simulink model "FW_IEEEIA"  (R2018b)
settings: Solver=ode45  StartTime=0.0  StopTime=30  FixedStep=Ts  RelTol=1e-4  EnableMultiTasking=on
InitFcn:
  | Ts = 1e-4;
  | 
  | 
  | Rs = 0.8975;
  | Ld = 15e-3;
  | Lq = 19e-3;
  | Pn = 3;
  | flux = 0.1764;
  | 
  | 
  | %ASR coef
  | kp_speed = 0.01;
  | ki_speed = 0.01*50;
  | 
  | kp_comp = 0.65;
  | ki_comp = 0.001*pi*kp_comp;
  | 
  | 
  | %FW coef
  | kpd_FW = 2;
  | kid_FW = 0.1;
  | 
  | 
  | %ACR coef
  | kp_cur = Lq*375;
  | ki_cur = Rs*375;
undefined symbols (not defined in the file or in its folder): DiscIntNeverNeededParam
libraries: powerlib x5, simulink x4, powerlib_extras x2
settings Model: Creator=SUN  LastModifiedBy=liangjin
settings SolverCC: ZeroCrossControl=DisableAll
settings DataIOCC: LimitDataPoints=on  SaveFormat=Array
settings OptimizationCC: ExpressionDepthLimit=2147483647  InitFltsAndDblsToZero=on  LifeSpan=inf
settings DebuggingCC: UnderspecifiedInitializationDetection=Classic  MergeDetectMultiDrivingBlocksExec=none  SolverPrmCheckMsg=warning  FcnCallInpInsideContextMsg=warning  StateNameClashWarn=warning  SFUnexpectedBacktrackingDiag=warning  SFNoUnconditionalDefaultTransitionDiag=warning  SFExecutionAtInitializationDiag=none
settings HardwareCC: ProdBitPerPointer=32  ProdBitPerSizeT=32  ProdBitPerPtrDiffT=32  ProdLargestAtomicFloat=None  ProdIntDivRoundTo=Undefined  ProdEndianess=Unspecified  ProdWordSize=32  ProdHWDeviceType=32-bit Generic
settings ModelReferenceCC: PropagateSignalLabelsOutOfModel=off
settings SFSimCC: SimUseLocalCustomCode=off
settings RTWCC: RTWUseLocalCustomCode=off
settings CodeAppCC: StateflowObjectComments=on
settings GRTTargetCC: TargetLangStandard=C89/C90 (ANSI)  CombineOutputUpdateFcns=off  GRTInterface=on
settings ConfigComp: CovMetricSettings=dw  CovHtmlReporting=on  CovSaveCumulativeToWorkspaceVar=on  CovSaveSingleToWorkspaceVar=on  CovExternalEMLEnable=off  CovSFcnEnable=off
settings SimscapeCC: SimscapeNormalizeSystem=off

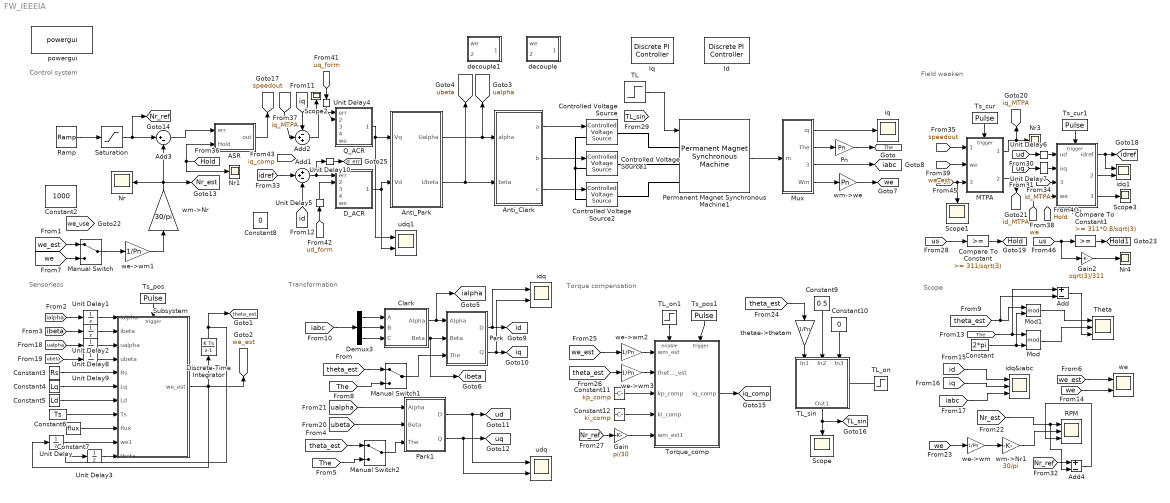
== system FW_IEEEIA ==
  note: Field weaken
  note: Control system
  note: Torque compensation
  note: Scope
  note: Transformation
  note: Sensorless
  ASR : Subsystem
  Add : Sum  Inputs=+-
  Add1 : Sum  Inputs=++-
  Add2 : Sum  Inputs=-++
  Add3 : Sum  Inputs=|+-
  Add4 : Sum  Inputs=+-
  Anti_Clark : Subsystem
  Anti_Park : Subsystem
  Clark : Subsystem
  Compare To Constant : simulink/Logic and Bit Operations/Compare To Constant  relop=>=  const=311/sqrt(3)  OutDataTypeStr=boolean
  Compare To Constant1 : simulink/Logic and Bit Operations/Compare To Constant  relop=>=  const=311*0.8/sqrt(3)  OutDataTypeStr=boolean
  Constant : Constant  Value=2*pi
  Constant10 : Constant  Value=0
  Constant11 : Constant  Value=kp_comp
  Constant12 : Constant  Value=ki_comp
  Constant2 : Constant  Value=1000
  Constant3 : Constant  Value=Rs
  Constant4 : Constant  Value=Lq
  Constant5 : Constant  Value=Ld
  Constant6 : Constant  Value=Ts
  Constant7 : Constant  Value=flux
  Constant8 : Constant  Value=0
  Constant9 : Constant  Value=0.5
  Controlled Voltage Source : powerlib/Electrical Sources/Controlled Voltage Source  Initialize=on  Source_Type=AC  Amplitude=0  Phase=0  Frequency=0  Measurements=Voltage
  Controlled Voltage Source1 : powerlib/Electrical Sources/Controlled Voltage Source  Initialize=on  Source_Type=AC  Amplitude=0  Phase=0  Frequency=0  Measurements=Voltage
  Controlled Voltage Source2 : powerlib/Electrical Sources/Controlled Voltage Source  Initialize=on  Source_Type=AC  Amplitude=0  Phase=0  Frequency=0  Measurements=Voltage
  D_ACR : Subsystem
  Demux3 : Demux  Outputs=3
  Discrete-Time Integrator : DiscreteIntegrator  gainval=1  SampleTime=Ts  ICPrevOutput=DiscIntNeverNeededParam  ICPrevScaledInput=DiscIntNeverNeededParam
  FW : Subsystem
  Gain : Gain  Gain=pi/30
  Gain2 : Gain  Gain=sqrt(3)/311
  Id : powerlib_extras/Discrete  Control Blocks/Discrete PI Controller  Kp=Ld*375  Ki=Rs*375  Par_Limits=[311*sqrt(1/3) -311*sqrt(1/3)]  Init=0  Ts=Ts
  Iq : powerlib_extras/Discrete  Control Blocks/Discrete PI Controller  Kp=Lq*375  Ki=Rs*375  Par_Limits=[311*sqrt(1/3) -311*sqrt(1/3)]  Init=0  Ts=Ts
  MTPA : Subsystem
  Manual Switch : ManualSwitch
  Manual Switch1 : ManualSwitch
  Manual Switch2 : ManualSwitch
  Mod : Math  Operator=mod  SaturateOnIntegerOverflow=on
  Mod1 : Math  Operator=mod  SaturateOnIntegerOverflow=on
  Mux : Subsystem
  Nr{,1,3..4} (4 alike) : Scope
  Park : Subsystem
  Park1 : Subsystem
  Permanent Magnet Synchronous Machine1 : powerlib/Machines/Permanent Magnet Synchronous Machine  NbPhases=3  FluxDistribution=Sinusoidal  RotorType=Salient-pole  MechanicalLoad=Torque Tm  PresetModel=No  ShowDetailedParameters=on  MeasurementBus=off  Resistance=0.8975  Inductance=8.5e-3  dqInductances=[15e-3,19e-3]  La=0.000835  MachineConstant=Flux linkage established by magnets (V.s)  Flux=0.1764  VoltageCst=95.9863  TorqueCst=0.7938  Flat=120  Mechanical=[0.000311 0.0000001 3 0]  PolePairs=3  InitialConditions=[0,0, 0,0]  InitialConditions5ph=[0 0 0 0 0 0]  TsPowergui=0  TsBlock=Ts  RefAngle=Aligned with phase A axis (original Park)
  Pn : Gain  Gain=Pn
  Q_ACR : Subsystem
  RPM : Scope  NumInputPorts=3
  Ramp : simulink/Sources/Ramp  slope=500  start=0  InitialOutput=0
  Saturation : Saturate  UpperLimit=6000  LowerLimit=-1000
  Scope{,1..3} (4 alike) : Scope
  Subsystem : Subsystem
  TL : Step  Time=5  After=0  SampleTime=Ts
  TL_on : Step  Time=5  SampleTime=0
  TL_on1 : Step  Time=5  SampleTime=0
  TL_sin : Subsystem
  Theta : Scope  NumInputPorts=3
  Torque_comp : Subsystem
  Ts_cur : DiscretePulseGenerator  PulseType=Time based  Period=Ts  PulseWidth=50
  Ts_cur1 : DiscretePulseGenerator  PulseType=Time based  Period=Ts  PulseWidth=50
  Ts_pos : DiscretePulseGenerator  PulseType=Time based  Period=Ts  PulseWidth=50
  Ts_pos1 : DiscretePulseGenerator  PulseType=Time based  Period=Ts  PulseWidth=50
  Unit Delay{,1..10} (11 alike) : UnitDelay  SampleTime=Ts
  decouple : Subsystem
  decouple1 : Subsystem
  idq : Scope  NumInputPorts=2
  idq&iabc : Scope  NumInputPorts=3
  idq1 : Scope  NumInputPorts=2
  iq : Scope
  powergui : powerlib/powergui  SimulationMode=Discrete  SampleTime=1e-5  frequency=60  Iterations=50  frequencyindice=0  Pbase=100e6  ErrMax=1e-4  UnitsV=kV  UnitsW=MW  buscounter=0  FunctionMessages=off  echomessages=off  EnableUseOfTLC=off  CurrentSourceSwitches=off  DisableSnubberDevices=off  DisableRonSwitches=off  DisableVfSwitches=off  DisplayEquations=off  SolverType=Tustin/Backward Euler (TBE)  Interpol=off  ExternalGateDelay=off  methode=off  Ts=100  x0status=blocks  SPID=off  SwTol=0  HookPort=off  RestoreLinks=warning  ResistiveCurrentMeasurement=off  Frange=[0:2:500]  Ylog=off  Xlog=on  ShowGrid=off  save=off  variable=ZData  structure=idq  ZoomFFT=off  StartTime=0.0  cycles=1  DisplayStyle=1  fundamental=60  FreqAxis=off  MaxFrequency=1000  frequencyindicesteady=1  RmsSteady=1  display=off
  thetae->thetam : Gain  Gain=1/Pn
  udq : Scope  NumInputPorts=2
  udq1 : Scope  NumInputPorts=2
  we : Scope  NumInputPorts=2
  we->wm{,1..3} (4 alike) : Gain  Gain=1/Pn
  wm->Nr : Gain  Gain=30/pi
  wm->Nr1 : Gain  Gain=30/pi
  wm->we : Gain  Gain=Pn
  tag scope: Hold1=global, Hold=global, Nr_est=global, Nr_ref=global, TL_sin=global, The=global, d_err=global, iabc=global, ialpha=global, ibeta=global, id=global, id_MTPA=global, idref=global, iq=global, iq_MTPA=global, iq_comp=global, speedout=global, theta_est=global, ualpha=global, ubeta=global, ud=global, uq=global, we=global, we_est=global, we_use=global
  wires:
  Permanent Magnet Synchronous Machine1/1 -> Mux/1(m)
  Add3/1 -> ASR/1(err)
  wm->Nr/1 -> [Nr_est], Add3/2, Nr/1
  Mux/1(iq) -> iq/1
  Mux/2(The) -> Pn/1
  Pn/1 -> [The]
  Mux/4(Wm) -> wm->we/1
  Mux/3(Iabc) -> [iabc]
  Clark/1(Alpha) -> [ialpha], Park/1(Alpha)
  Demux3/1 -> Clark/1(A)
  Demux3/2 -> Clark/2(B)
  Demux3/3 -> Clark/3(C)
  Clark/2(Beta) -> Park/2(Beta), [ibeta]
  Anti_Clark/2(b) -> Controlled Voltage Source1/1
  Anti_Clark/3(c) -> Controlled Voltage Source2/1
  Constant/1 -> Mod1/2, Mod/2
  Mod/1 -> Theta/2
  wm->we/1 -> [we]
  Ramp/1 -> Saturation/1
  we->wm1/1 -> wm->Nr/1
  Anti_Park/1(Ualpha) -> Anti_Clark/1(alpha), [ualpha]
  Anti_Park/2(Ubeta) -> Anti_Clark/2(beta), [ubeta]
  [we_est] -> we/1
  [we_est] -> Manual Switch/1
  [we] -> Manual Switch/2
  [theta_est] -> Manual Switch1/1
  [The] -> Manual Switch1/2
  Park/1(D) -> idq/1, [id]
  Park/2(Q) -> [iq], idq/2
  [The] -> Add/1, Mod/1
  [id] -> idq&iabc/1
  [iq] -> idq&iabc/2
  [iabc] -> idq&iabc/3
  [id] -> Add1/3
  [iq] -> Add2/1
  [The] -> Manual Switch2/2
  [theta_est] -> Manual Switch2/1
  [ubeta] -> Park1/2(Beta)
  [ualpha] -> Park1/1(Alpha)
  Park1/1(D) -> [ud], udq/1
  Park1/2(Q) -> udq/2, [uq]
  Constant3/1 -> Subsystem/5(Rs)
  Constant4/1 -> Subsystem/6(Lq)
  Constant5/1 -> Subsystem/7(Ld)
  Constant6/1 -> Subsystem/8(Ts)
  Constant7/1 -> Subsystem/9(flux)
  Unit Delay/1 -> Subsystem/10(we1)
  Ts_pos/1 -> Subsystem/Trigger
  Unit Delay3/1 -> Subsystem/11(theta)
  [theta_est] -> Add/2, Mod1/1
  Mod1/1 -> Theta/1
  [iabc] -> Demux3/1
  Discrete-Time Integrator/1 -> Unit Delay3/1, [theta_est]
  Anti_Clark/1(a) -> Controlled Voltage Source/1
  [we] -> we->wm/1
  we->wm/1 -> wm->Nr1/1
  wm->Nr1/1 -> RPM/2
  [Nr_est] -> Add4/2, RPM/1
  Ts_cur/1 -> MTPA/Trigger
  [we] -> we/2
  [theta_est] -> thetae->thetam/1
  thetae->thetam/1 -> TL_sin/1(In1)
  Constant9/1 -> TL_sin/2(In2)
  Constant10/1 -> TL_sin/3(In3)
  TL_on/1 -> TL_sin/Enable
  TL_sin/1(Out1) -> [TL_sin], Scope/1
  we->wm2/1 -> Torque_comp/1(wm_est)
  we->wm3/1 -> Torque_comp/2(thetam_est)
  Constant11/1 -> Torque_comp/3(kp_comp)
  Constant12/1 -> Torque_comp/4(ki_comp)
  Torque_comp/1(iq_comp) -> [iq_comp]
  [Nr_ref] -> Gain/1
  Gain/1 -> Torque_comp/5(wm_est1)
  Ts_pos1/1 -> Torque_comp/Trigger
  TL_on1/1 -> Torque_comp/Enable
  [we_est] -> we->wm2/1
  [theta_est] -> we->wm3/1
  Ts_cur1/1 -> FW/Trigger
  [speedout] -> MTPA/1(speedout)
  Add/1 -> Theta/3
  MTPA/1(iq_MTPA) -> Nr3/1, [iq_MTPA]
  MTPA/2(id_MTPA) -> [id_MTPA]
  [idref] -> Add1/2
  [Nr_ref] -> Add4/1
  Add4/1 -> RPM/3
  [id_MTPA] -> FW/3(id_MTPA)
  Saturation/1 -> Add3/1, [Nr_ref]
  ASR/1(out) -> [speedout]
  [iq_MTPA] -> Add2/2
  [us] -> Compare To Constant/1
  Compare To Constant/1 -> [Hold]
  [we] -> FW/4(we)
  [we_est] -> MTPA/2(we)
  FW/1(idref) -> [idref], idq1/1
  [uq_form] -> Unit Delay4/1
  Unit Delay4/1 -> Q_ACR/2(uq_form)
  [ud_form] -> Unit Delay5/1
  Unit Delay5/1 -> D_ACR/2(ud_form)
  FW/2(piout) -> idq1/2
  Add2/1 -> Scope2/1, Q_ACR/1(err)
  Add1/1 -> Unit Delay10/1, D_ACR/1(err)
  Q_ACR/1(iqout) -> udq1/1, Anti_Park/1(Vq)
  D_ACR/1(idout) -> Anti_Park/2(Vd), udq1/2
  [ud] -> Unit Delay6/1
  Unit Delay6/1 -> FW/1(ud)
  [uq] -> Unit Delay7/1
  Unit Delay7/1 -> FW/2(uq)
  [us] -> Gain2/1, Compare To Constant1/1
  Gain2/1 -> Nr4/1
  Compare To Constant1/1 -> [Hold1]
  Subsystem/1(we_est) -> [we_est], Discrete-Time Integrator/1, Unit Delay/1
  [ualpha] -> Unit Delay8/1
  [ubeta] -> Unit Delay9/1
  [ialpha] -> Unit Delay1/1
  [ibeta] -> Unit Delay2/1
  Manual Switch/1 -> we->wm1/1
  Unit Delay1/1 -> Subsystem/1(ialpha)
  Unit Delay2/1 -> Subsystem/2(ibeta)
  Unit Delay8/1 -> Subsystem/3(ualpha)
  Unit Delay9/1 -> Subsystem/4(ubeta)
  Manual Switch2/1 -> Park1/3(The)
  Manual Switch1/1 -> Park/3(The)
  TL/1 -> Permanent Magnet Synchronous Machine1/1
  [Hold] -> ASR/2(Hold), Nr1/1
  [d_err] -> Scope1/1, MTPA/3(d_err)
  Unit Delay10/1 -> [d_err]
  FW/3(id_mtpa) -> Scope3/1
  connections:
  Controlled Voltage Source/LConn1 -- Controlled Voltage Source2/LConn1 -- Controlled Voltage Source1/LConn1
  Controlled Voltage Source/RConn1 -- Permanent Magnet Synchronous Machine1/LConn1
  Controlled Voltage Source1/RConn1 -- Permanent Magnet Synchronous Machine1/LConn2
  Controlled Voltage Source2/RConn1 -- Permanent Magnet Synchronous Machine1/LConn3

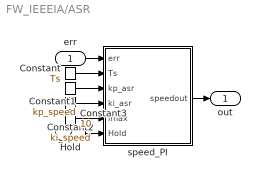
== system FW_IEEEIA/ASR ==
  err : Inport
  Hold : Inport  Port=2
  Constant : Constant  Value=Ts
  Constant1 : Constant  Value=kp_speed
  Constant2 : Constant  Value=ki_speed
  Constant3 : Constant  Value=10
  speed_PI : MATLAB Function  TreatAsAtomicUnit=on
  out : Outport
  wires:
  err/1 -> speed_PI/1(err)
  Constant3/1 -> speed_PI/5(imax)
  Constant2/1 -> speed_PI/4(ki_asr)
  Constant/1 -> speed_PI/2(Ts)
  Constant1/1 -> speed_PI/3(kp_asr)
  Hold/1 -> speed_PI/6(Hold)
  speed_PI/1(speedout) -> out/1

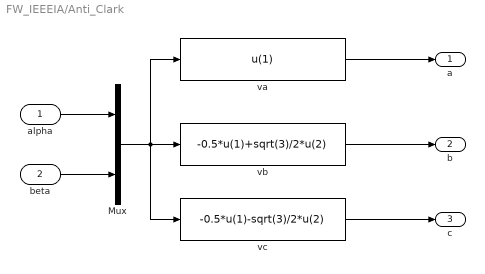
== system FW_IEEEIA/Anti_Clark ==
  alpha : Inport
  beta : Inport  Port=2
  Mux : Mux  Inputs=2
  va : Fcn  Expr=u(1)
  vb : Fcn  Expr=-0.5*u(1)+sqrt(3)/2*u(2)
  vc : Fcn  Expr=-0.5*u(1)-sqrt(3)/2*u(2)
  a : Outport
  b : Outport  Port=2
  c : Outport  Port=3
  wires:
  va/1 -> a/1
  beta/1 -> Mux/2
  alpha/1 -> Mux/1
  Mux/1 -> vc/1, vb/1, va/1
  vb/1 -> b/1
  vc/1 -> c/1

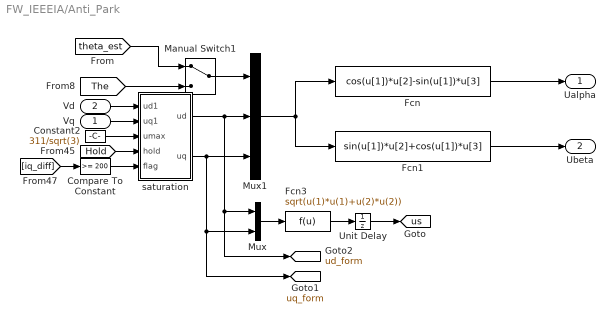
== system FW_IEEEIA/Anti_Park ==
  Vq : Inport
  Vd : Inport  Port=2
  Compare To Constant : simulink/Logic and Bit Operations/Compare To Constant  relop=>=  const=200  OutDataTypeStr=boolean
  Constant2 : Constant  Value=311/sqrt(3)
  Fcn : Fcn  Expr=cos(u[1])*u[2]-sin(u[1])*u[3]
  Fcn1 : Fcn  Expr=sin(u[1])*u[2]+cos(u[1])*u[3]
  Fcn3 : Fcn  Expr=sqrt(u(1)*u(1)+u(2)*u(2))
  Manual Switch1 : ManualSwitch
  Mux : Mux  Inputs=2
  Mux1 : Mux  Inputs=3
  Unit Delay : UnitDelay  SampleTime=-1
  saturation : MATLAB Function  TreatAsAtomicUnit=on
  Ualpha : Outport
  Ubeta : Outport  Port=2
  tag scope: ud_form=global, uq_form=global, us=global
  wires:
  Fcn1/1 -> Ubeta/1
  Fcn/1 -> Ualpha/1
  Mux1/1 -> Fcn/1, Fcn1/1
  [The] -> Manual Switch1/2
  [theta_est] -> Manual Switch1/1
  Vq/1 -> saturation/2(uq1)
  Vd/1 -> saturation/1(ud1)
  Constant2/1 -> saturation/3(umax)
  Mux/1 -> Fcn3/1
  Fcn3/1 -> Unit Delay/1
  Unit Delay/1 -> [us]
  saturation/1(ud) -> Mux1/2, [ud_form], Mux/1
  saturation/2(uq) -> [uq_form], Mux/2, Mux1/3
  [Hold] -> saturation/4(hold)
  [iq_diff] -> Compare To Constant/1
  Manual Switch1/1 -> Mux1/1
  Compare To Constant/1 -> saturation/5(flag)

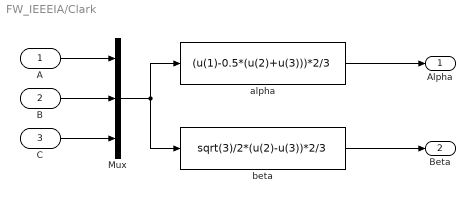
== system FW_IEEEIA/Clark ==
  A : Inport
  B : Inport  Port=2
  C : Inport  Port=3
  Mux : Mux  Inputs=3
  alpha : Fcn  Expr=(u(1)-0.5*(u(2)+u(3)))*2/3
  beta : Fcn  Expr=sqrt(3)/2*(u(2)-u(3))*2/3
  Alpha : Outport
  Beta : Outport  Port=2
  wires:
  alpha/1 -> Alpha/1
  B/1 -> Mux/2
  C/1 -> Mux/3
  A/1 -> Mux/1
  Mux/1 -> beta/1, alpha/1
  beta/1 -> Beta/1

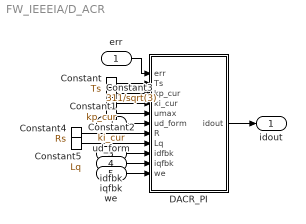
== system FW_IEEEIA/D_ACR ==
  err : Inport
  ud_form : Inport  Port=2
  idfbk : Inport  Port=3
  iqfbk : Inport  Port=4
  we : Inport  Port=5
  Constant : Constant  Value=Ts
  Constant1 : Constant  Value=kp_cur
  Constant2 : Constant  Value=ki_cur
  Constant3 : Constant  Value=311/sqrt(3)
  Constant4 : Constant  Value=Rs
  Constant5 : Constant  Value=Lq
  DACR_PI : MATLAB Function  TreatAsAtomicUnit=on
  idout : Outport
  wires:
  err/1 -> DACR_PI/1(err)
  Constant3/1 -> DACR_PI/5(umax)
  Constant2/1 -> DACR_PI/4(ki_cur)
  Constant/1 -> DACR_PI/2(Ts)
  Constant1/1 -> DACR_PI/3(kp_cur)
  ud_form/1 -> DACR_PI/6(ud_form)
  DACR_PI/1(idout) -> idout/1
  Constant4/1 -> DACR_PI/7(R)
  Constant5/1 -> DACR_PI/8(Lq)
  idfbk/1 -> DACR_PI/9(idfbk)
  iqfbk/1 -> DACR_PI/10(iqfbk)
  we/1 -> DACR_PI/11(we)

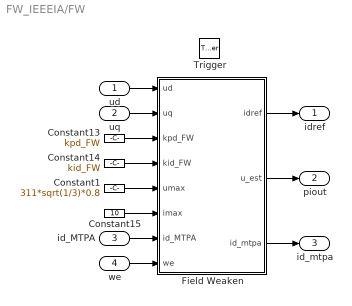
== system FW_IEEEIA/FW ==
  ud : Inport
  uq : Inport  Port=2
  id_MTPA : Inport  Port=3
  we : Inport  Port=4
  Trigger : TriggerPort  VariantControl=Variant  PortDimensions=1
  Constant1 : Constant  Value=311*sqrt(1/3)*0.8
  Constant13 : Constant  Value=kpd_FW
  Constant14 : Constant  Value=kid_FW
  Constant15 : Constant  Value=10
  Field Weaken : MATLAB Function  TreatAsAtomicUnit=on
  idref : Outport
  piout : Outport  Port=2
  id_mtpa : Outport  Port=3
  wires:
  Constant13/1 -> Field Weaken/3(kpd_FW)
  Constant15/1 -> Field Weaken/6(imax)
  Constant14/1 -> Field Weaken/4(kid_FW)
  uq/1 -> Field Weaken/2(uq)
  Constant1/1 -> Field Weaken/5(umax)
  ud/1 -> Field Weaken/1(ud)
  id_MTPA/1 -> Field Weaken/7(id_MTPA)
  we/1 -> Field Weaken/8(we)
  Field Weaken/2(u_est) -> piout/1
  Field Weaken/1(idref) -> idref/1
  Field Weaken/3(id_mtpa) -> id_mtpa/1

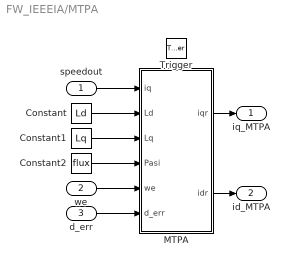
== system FW_IEEEIA/MTPA ==
  speedout : Inport
  we : Inport  Port=2
  d_err : Inport  Port=3
  Trigger : TriggerPort  VariantControl=Variant  PortDimensions=1
  Constant : Constant  Value=Ld
  Constant1 : Constant  Value=Lq
  Constant2 : Constant  Value=flux
  MTPA : MATLAB Function  TreatAsAtomicUnit=on
  iq_MTPA : Outport
  id_MTPA : Outport  Port=2
  wires:
  MTPA/2(idr) -> id_MTPA/1
  MTPA/1(iqr) -> iq_MTPA/1
  speedout/1 -> MTPA/1(iq)
  Constant/1 -> MTPA/2(Ld)
  Constant1/1 -> MTPA/3(Lq)
  Constant2/1 -> MTPA/4(Pasi)
  we/1 -> MTPA/5(we)
  d_err/1 -> MTPA/6(d_err)

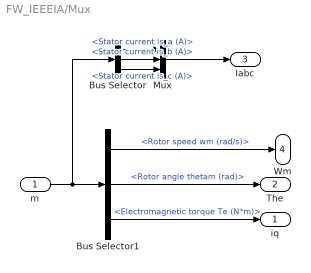
== system FW_IEEEIA/Mux ==
  m : Inport
  Bus Selector : BusSelector  OutputSignals=Stator current is_a (A),Stator current is_b (A),Stator current is_c (A)
  Bus Selector1 : BusSelector  OutputSignals=Rotor speed wm (rad/s),Rotor angle thetam (rad),Electromagnetic torque Te (N*m)
  Mux : Mux  Inputs=3
  iq : Outport
  The : Outport  Port=2
  Iabc : Outport  Port=3
  Wm : Outport  Port=4
  wires:
  Bus Selector1/1 -> Wm/1  "<Rotor speed wm (rad/s)>"
  Bus Selector1/2 -> The/1  "<Rotor angle thetam (rad)>"
  Bus Selector1/3 -> iq/1  "<Electromagnetic torque Te (N*m)>"
  m/1 -> Bus Selector/1, Bus Selector1/1
  Bus Selector/2 -> Mux/2  "<Stator current is_b (A)>"
  Bus Selector/3 -> Mux/3  "<Stator current is_c (A)>"
  Bus Selector/1 -> Mux/1  "<Stator current is_a (A)>"
  Mux/1 -> Iabc/1

== system FW_IEEEIA/Park ==
  Alpha : Inport
  Beta : Inport  Port=2
  The : Inport  Port=3
  Mux : Mux  Inputs=3
  d : Fcn  Expr=u(1)*cos(u(3))+u(2)*sin(u(3))
  q : Fcn  Expr=-u(1)*sin(u(3))+u(2)*cos(u(3))
  D : Outport
  Q : Outport  Port=2
  wires:
  d/1 -> D/1
  Beta/1 -> Mux/2
  Alpha/1 -> Mux/1
  Mux/1 -> q/1, d/1
  q/1 -> Q/1
  The/1 -> Mux/3

== system FW_IEEEIA/Park1 ==
  Alpha : Inport
  Beta : Inport  Port=2
  The : Inport  Port=3
  Mux : Mux  Inputs=3
  d : Fcn  Expr=u(1)*cos(u(3))+u(2)*sin(u(3))
  q : Fcn  Expr=-u(1)*sin(u(3))+u(2)*cos(u(3))
  D : Outport
  Q : Outport  Port=2
  wires:
  d/1 -> D/1
  Beta/1 -> Mux/2
  Alpha/1 -> Mux/1
  Mux/1 -> q/1, d/1
  q/1 -> Q/1
  The/1 -> Mux/3

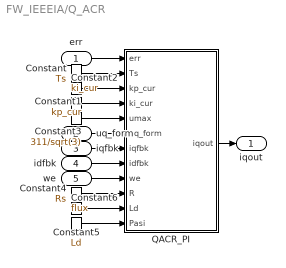
== system FW_IEEEIA/Q_ACR ==
  err : Inport
  uq_form : Inport  Port=2
  iqfbk : Inport  Port=3
  idfbk : Inport  Port=4
  we : Inport  Port=5
  Constant : Constant  Value=Ts
  Constant1 : Constant  Value=kp_cur
  Constant2 : Constant  Value=ki_cur
  Constant3 : Constant  Value=311/sqrt(3)
  Constant4 : Constant  Value=Rs
  Constant5 : Constant  Value=Ld
  Constant6 : Constant  Value=flux
  QACR_PI : MATLAB Function  TreatAsAtomicUnit=on
  iqout : Outport
  wires:
  err/1 -> QACR_PI/1(err)
  Constant3/1 -> QACR_PI/5(umax)
  Constant2/1 -> QACR_PI/4(ki_cur)
  Constant/1 -> QACR_PI/2(Ts)
  Constant1/1 -> QACR_PI/3(kp_cur)
  uq_form/1 -> QACR_PI/6(uq_form)
  QACR_PI/1(iqout) -> iqout/1
  Constant4/1 -> QACR_PI/10(R)
  Constant5/1 -> QACR_PI/11(Ld)
  Constant6/1 -> QACR_PI/12(Pasi)
  we/1 -> QACR_PI/9(we)
  idfbk/1 -> QACR_PI/8(idfbk)
  iqfbk/1 -> QACR_PI/7(iqfbk)

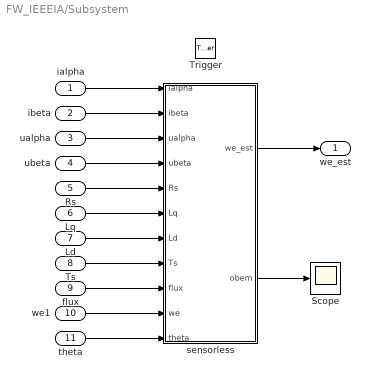
== system FW_IEEEIA/Subsystem ==
  ialpha : Inport
  ibeta : Inport  Port=2
  ualpha : Inport  Port=3
  ubeta : Inport  Port=4
  Rs : Inport  Port=5
  Lq : Inport  Port=6
  Ld : Inport  Port=7
  Ts : Inport  Port=8
  flux : Inport  Port=9
  we1 : Inport  Port=10
  theta : Inport  Port=11
  Trigger : TriggerPort  VariantControl=Variant  PortDimensions=1
  Scope : Scope
  sensorless : MATLAB Function  TreatAsAtomicUnit=on
  we_est : Outport
  wires:
  ualpha/1 -> sensorless/3(ualpha)
  Ts/1 -> sensorless/8(Ts)
  flux/1 -> sensorless/9(flux)
  ialpha/1 -> sensorless/1(ialpha)
  sensorless/1(we_est) -> we_est/1
  Lq/1 -> sensorless/6(Lq)
  ubeta/1 -> sensorless/4(ubeta)
  ibeta/1 -> sensorless/2(ibeta)
  Rs/1 -> sensorless/5(Rs)
  Ld/1 -> sensorless/7(Ld)
  we1/1 -> sensorless/10(we)
  theta/1 -> sensorless/11(theta)
  sensorless/2(obem) -> Scope/1

== system FW_IEEEIA/TL_sin ==
  In1 : Inport
  In2 : Inport  Port=2
  In3 : Inport  Port=3
  Enable : EnablePort
  MATLAB Function : MATLAB Function  TreatAsAtomicUnit=on
  Out1 : Outport
  wires:
  In1/1 -> MATLAB Function/1(Theta_m)
  MATLAB Function/1(TL) -> Out1/1
  In3/1 -> MATLAB Function/3(Theta0)
  In2/1 -> MATLAB Function/2(Amp)

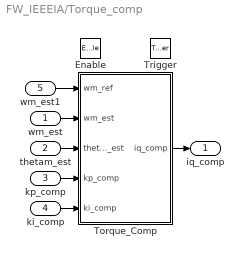
== system FW_IEEEIA/Torque_comp ==
  wm_est : Inport
  thetam_est : Inport  Port=2
  kp_comp : Inport  Port=3
  ki_comp : Inport  Port=4
  wm_est1 : Inport  Port=5
  Enable : EnablePort
  Trigger : TriggerPort  VariantControl=Variant  PortDimensions=1
  Torque_Comp : MATLAB Function  TreatAsAtomicUnit=on
  iq_comp : Outport
  wires:
  Torque_Comp/1(iq_comp) -> iq_comp/1
  kp_comp/1 -> Torque_Comp/4(kp_comp)
  wm_est/1 -> Torque_Comp/2(wm_est)
  ki_comp/1 -> Torque_Comp/5(ki_comp)
  wm_est1/1 -> Torque_Comp/1(wm_ref)
  thetam_est/1 -> Torque_Comp/3(thetam_est)

== system FW_IEEEIA/decouple ==
  we : Inport
  iqref : Inport  Port=2
  Constant : Constant  Value=Lq
  decouple : MATLAB Function  TreatAsAtomicUnit=on
  udq : Outport
  wires:
  we/1 -> decouple/1(we)
  Constant/1 -> decouple/2(Lq)
  iqref/1 -> decouple/3(iqref)
  decouple/1(udq) -> udq/1

== system FW_IEEEIA/decouple1 ==
  we : Inport
  idref : Inport  Port=2
  Constant : Constant  Value=Lq
  Constant1 : Constant  Value=flux
  decouple : MATLAB Function  TreatAsAtomicUnit=on
  uqd : Outport
  wires:
  decouple/1(uqd) -> uqd/1
  idref/1 -> decouple/3(idref)
  Constant/1 -> decouple/2(Ld)
  we/1 -> decouple/1(we)
  Constant1/1 -> decouple/4(Pasi)

== matlab function FW_IEEEIA/MTPA/MTPA ==
  data: iqr output; iq input; idr output; Ld input; Lq input; Pasi input; we input; d_err input
function [iqr,idr] = MTPA(iq,Ld,Lq,Pasi,we,d_err)

persistent id1 iq1 iq_sat;

if isempty(id1)
    id1=0;iq1=0;iq_sat=0;
end

iq_sat = 16.82-0.01108*we+0.000002*we*we;

iq1 = iq;

if(iq1<0)
    iq1=0;
% elseif(iq1>iq_sat)
%     iq1=iq_sat;
end

id1 = iq1*iq1*(Ld-Lq)/Pasi;
% id1 = 0;

idr = id1;
iqr = iq1;

== matlab function FW_IEEEIA/Subsystem/sensorless ==
  data: ialpha input; we_est output; ibeta input; ualpha input; ubeta input; Rs input; Lq input; Ld input; Ts input; flux input; we input; theta input; obem output

function [we_est, obem]  = sensorless(ialpha,ibeta,ualpha,ubeta,Rs,Lq,Ld,Ts,flux,we,theta)

persistent id2 iq2 delta_id delta_iq bemf we1 flag;

if isempty(id2)
    id2=0;iq2=0;delta_id=0;delta_iq=0;bemf=0;we1=0;flag=0;obem=0;
end

ud= cos(theta)*ualpha+sin(theta)*ubeta;
uq=-sin(theta)*ualpha+cos(theta)*ubeta;
id1= cos(theta)*ialpha+sin(theta)*ibeta;
iq1=-sin(theta)*ialpha+cos(theta)*ibeta;

if(bemf < 0)
    flag = 1;
end

we1 = we1+0.715*(we-we1);
temp1 = ud-id2*Rs;
temp1 = temp1+we1*Lq*iq2;
temp1 = temp1*Ts/Ld + id2;
delta_id = delta_id+0.125*((temp1-id1)-delta_id);

temp2 = uq-iq2*Rs;
temp2 = temp2-we1*Ld*id2;
temp2 = temp2-bemf;
temp2 = Ts*temp2/Lq+iq2;
delta_iq = delta_iq+0.5*((temp2-iq1)-delta_iq);

bemf = bemf+delta_iq*Lq/Ts;
if(flag)
    we_est = (bemf+delta_id*Ld/Ts)/flux;
else
    we_est = (bemf-delta_id*Ld/Ts)/flux;
end
obem = bemf;
id2 = id1;
iq2 = iq1;

== matlab function FW_IEEEIA/TL_sin/MATLAB Function ==
  data: Theta_m input; TL output; Amp input; Theta0 input
function TL = fcn(Theta_m,Amp,Theta0)
if isempty(Theta_m)
    Theta_m=0;Amp=0;Theta0=0;TL=0;
end
TL = Amp*sin(Theta_m+Theta0);

== matlab function FW_IEEEIA/Torque_comp/Torque_Comp ==
  data: wm_ref input; iq_comp output; wm_est input; thetam_est input; kp_comp input; ki_comp input
function iq_comp = Torque_Comp(wm_ref,wm_est,thetam_est,kp_comp,ki_comp)

persistent Te temp1 temp2 up ui1 ui2 out1 out2 comp1_fbk comp2_fbk comp1_ref comp2_ref;

if isempty(temp1)
    Te=0; temp1=0; temp2=0; up=0; ui1=0; ui2=0; out1=0; out2=0; iq_comp=0; 
    comp1_fbk=0; comp2_fbk=0; comp1_ref=0; comp2_ref=0;
end

%calc comp sin value
Te = wm_ref-wm_est;
temp1 = Te*sin(thetam_est);
comp1_fbk = 0;
if (wm_ref < 10)
    comp1_ref = 0;
else
    comp1_ref = temp1;
end
up = comp1_ref - comp1_fbk;
ui1 = ui1 + ki_comp*up;
out1 = kp_comp*up + ui1;

%calc comp cos value
temp2 = Te*cos(thetam_est);
comp2_fbk = 0;
if (wm_ref < 10)
    comp2_ref = 0;
else
    comp2_ref = temp2;
end
up = comp2_ref - comp2_fbk;
ui2 = ui2 + ki_comp*up;
out2 = kp_comp*up + ui2;

iq_comp = out1*sin(thetam_est) + out2*cos(thetam_est);

if (iq_comp > 10)
    iq_comp = 10;
elseif (iq_comp < -10)
    iq_comp = -10;
end

== matlab function FW_IEEEIA/FW/Field Weaken ==
  data: idref output; ud input; uq input; kpd_FW input; kid_FW input; umax input; imax input; id_MTPA input; we input; u_est output; id_mtpa output
function [idref,u_est,id_mtpa]   = Fieldweaken(ud,uq,kpd_FW,kid_FW,umax,imax,id_MTPA,we)

persistent us uout ui up id1 id_sat;

isempty (us)
    us=0;ui=0;id1=0;uout=0;id_sat=0;

us = sqrt(ud.^2+uq.^2);

id_sat = 5.385-0.01537*we+0.000004*we*we;

    up = umax - us;
    ui = ui+up*kid_FW;
    uout = kpd_FW*up+ui;
    
    id1 = id1+id_MTPA;
    
if (id1<-imax)
    id1 = -imax;
elseif (id1>0)
    id1 = 0;
end

u_est = uout; 
idref = id1;
id_mtpa = id_MTPA;

== matlab function FW_IEEEIA/ASR/speed_PI ==
  data: err input; speedout output; Ts input; kp_asr input; ki_asr input; imax input; Hold input
function speedout   = speed_PI(err,Ts,kp_asr,ki_asr,imax,Hold)

persistent up ui temp temp1;

if isempty(up)
    up=0;ui=0;temp=0;temp1=0;
end

if (Hold)
    temp = temp1;
else
    ui = ui+err*Ts*ki_asr;
    up = err*kp_asr;
    temp = ui+up;
end
if(temp>=imax)
    temp1 = imax;
elseif(temp<-imax)
    temp1 =  -imax;
else
    temp1 = temp;
end
ui = temp1-up;
speedout = temp1;

== matlab function FW_IEEEIA/Anti_Park/saturation ==
  data: ud1 input; ud output; uq1 input; umax input; uq output; hold input; flag input
function [ud,uq] = saturation(ud1,uq1,umax,hold,flag)

persistent us uq2 ud2;

if isempty(us)
    us=0;uq2=0;ud2=0;
end
us = sqrt(ud1.^2+uq1.^2);
% ud2 = ud1;
% if(us>=umax)
%     uq2 = sqrt(umax.^2-ud1.^2);
% else
%     uq2 = uq1;
% end

if( us>=umax)
%     uq2 = umax*uq1/us;
%     ud2 = umax*ud1/us;
    uq2 = sqrt(umax.^2-ud1.^2);
    ud2 = ud1;
else
    uq2 = uq1;
    ud2 = ud1;
end
% if(hold && (uq2>137))
%     uq2 = 137;
%     ud2 = sqrt(umax.^2-uq2.^2);
% end

ud = ud2;
uq = uq2;

== matlab function FW_IEEEIA/Q_ACR/QACR_PI ==
  data: err input; iqout output; Ts input; kp_cur input; ki_cur input; umax input; uq_form input; iqfbk input; idfbk input; we input; R input; Ld input; Pasi input
function iqout  = QACR_PI(err,Ts,kp_cur,ki_cur,umax,uq_form,iqfbk,idfbk,we,R,Ld,Pasi)

persistent up ui temp uq_sat;

if isempty(up)
    up=0;ui=0;temp=0;uq_sat=0;
end
% uq_sat = R*iqfbk+1885*Ld*idfbk+1885*Pasi;
ui = uq_form-up;
ui = ui+err*Ts*ki_cur;
up = err*kp_cur;
if(ui>umax)
    ui = umax;
elseif(ui<-umax)
    ui =  -umax;
end
temp = ui+up;
if(temp>umax)
    temp = umax;
elseif(temp<-umax)
    temp =  -umax;
end

iqout = temp;

== matlab function FW_IEEEIA/D_ACR/DACR_PI ==
  data: err input; idout output; Ts input; kp_cur input; ki_cur input; umax input; ud_form input; R input; Lq input; idfbk input; iqfbk input; we input
function idout  = DACR_PI(err,Ts,kp_cur,ki_cur,umax,ud_form,R,Lq,idfbk,iqfbk,we)

persistent up ui temp ud_sat;

if isempty(up)
    up=0;ui=0;temp=0;ud_sat=0;
end

ud_sat = R*idfbk-we*Lq*iqfbk;

ui = ud_form-up;
ui = ui+err*Ts*ki_cur;
up = err*kp_cur;
if(ui>umax)
    ui = umax;
elseif(ui<-umax)
    ui =  -umax;
end
temp = ui+up;
if(temp>umax)
    temp = umax;
elseif(temp<-umax)
    temp =  -umax;
end
% if(temp>0)
%     temp = 0;
% elseif(temp>ud_sat)
%     temp =  ud_sat;
% end

idout = temp;

== matlab function FW_IEEEIA/decouple/decouple ==
  data: we input; udq output; Lq input; iqref input
function udq  = decouple(we,Lq,iqref)

udq = we*Lq*iqref;

== matlab function FW_IEEEIA/decouple1/decouple ==
  data: we input; uqd output; Ld input; idref input; Pasi input
function uqd  = decouple(we,Ld,idref,Pasi)

uqd = we*Ld*idref+we*Pasi;
